simulink model "twoCnts"  (R2025b)
settings: Solver=FixedStepDiscrete  StartTime=0.0  StopTime=Inf  RelTol=1e-3
settings Model: Creator=Soochan Kim  LastModifiedBy=Soochan Kim
settings OptimizationCC: BlockReduction=off  ConditionallyExecuteInputs=off  DefaultParameterBehavior=Inlined
settings DebuggingCC: AlgebraicLoopMsg=error
settings HardwareCC: ProdBitPerPointer=32.0  ProdBitPerSizeT=32.0  ProdBitPerPtrDiffT=32.0  ProdLargestAtomicFloat=None  ProdIntDivRoundTo=Undefined  ProdEndianess=Unspecified  ProdWordSize=32.0  ProdHWDeviceType=ASIC/FPGA->ASIC/FPGA  TargetBitPerPointer=64.0  TargetBitPerSizeT=64.0  TargetBitPerPtrDiffT=64.0  TargetLongLongMode=on  TargetIntDivRoundTo=Zero  TargetEndianess=LittleEndian  TargetWordSize=64.0  TargetHWDeviceType=Custom Processor->MATLAB Host Computer  ProdEqTarget=off

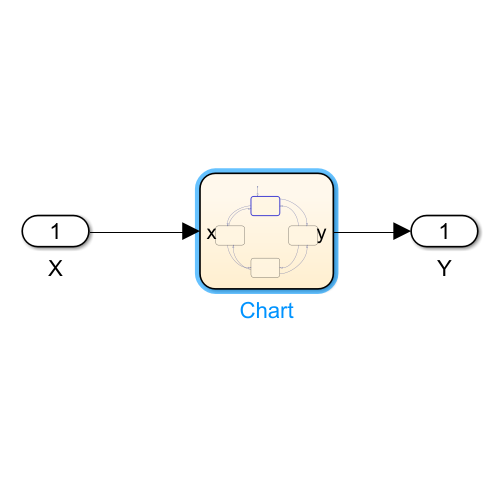
[thumbnail: Simulink's stored preview of the top-level diagram]
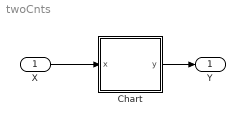
== system twoCnts ==
  X : Inport  OutDataTypeStr=boolean
  Chart : Stateflow chart  TreatAsAtomicUnit=on
  Y : Outport
  wires:
  X/1 -> Chart/1(x)
  Chart/1(y) -> Y/1

== stateflow chart twoCnts/Chart ==
  settings: executeAtInitialization=1
  state S0
    y=0;
  state S02
    y=1;
  state S01
    y=3;
  state S03
    y=2;
  (default) -> S0
  S0 -> S01 [order 2] : [x==0]
  S01 -> S0 [order 1] : [x==1]
  S0 -> S02 [order 1] : [x==1]
  S02 -> S0 [order 2] : [x==0]
  S02 -> S03 [order 1] : [x==1]
  S03 -> S02 [order 2] : [x==0]
  S03 -> S01 [order 1] : [x==1]
  S01 -> S03 [order 2] : [x==0]
  data: x input boolean; y output fixdt(1,2,0)
